simulink model "param_monitor"  (R2021a)
settings: Solver=VariableStepAuto  StartTime=0.0  StopTime=10.0  RelTol=1e-3
values from neighbouring files (symbols this model uses):
  sys_regs = 1    [motor_data.sldd]
settings Model: DataDictionary=motor_data.sldd  Creator=Litao  LastModifiedBy=Litao

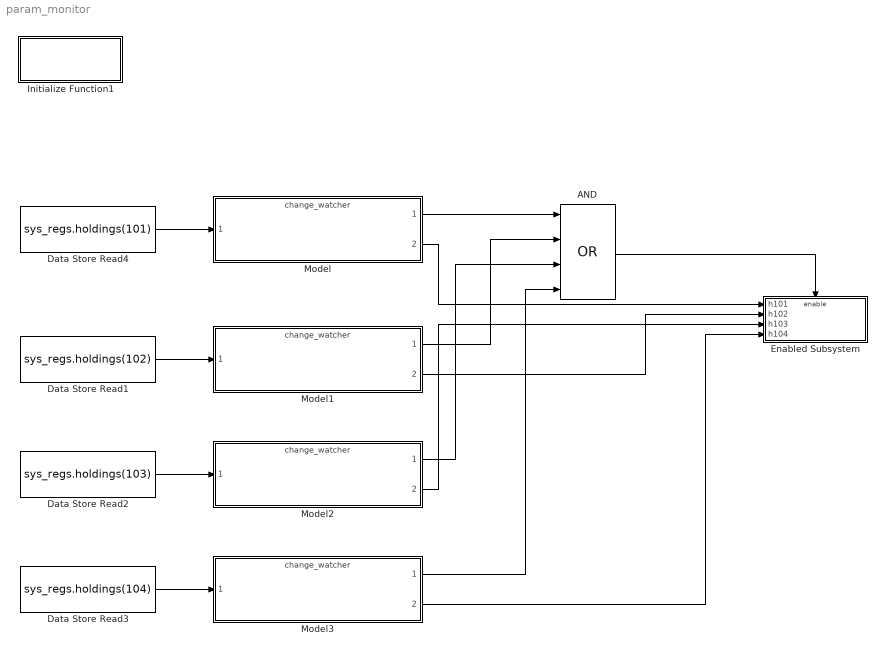
== system param_monitor ==
  AND : Logic  Operator=OR  Inputs=4  AllPortsSameDT=off  OutDataTypeStr=boolean
  Data Store Read1 : DataStoreRead  DataStoreName=sys_regs  DataStoreElements=sys_regs.holdings(102)  IndexOptions=Index vector (dialog)  Indices=1  OutputSizes=1
  Data Store Read2 : DataStoreRead  DataStoreName=sys_regs  DataStoreElements=sys_regs.holdings(103)  IndexOptions=Index vector (dialog)  Indices=1  OutputSizes=1
  Data Store Read3 : DataStoreRead  DataStoreName=sys_regs  DataStoreElements=sys_regs.holdings(104)  IndexOptions=Index vector (dialog)  Indices=1  OutputSizes=1
  Data Store Read4 : DataStoreRead  DataStoreName=sys_regs  DataStoreElements=sys_regs.holdings(101)  IndexOptions=Index vector (dialog)  Indices=1  OutputSizes=1
  Enabled Subsystem : Subsystem  TreatAsAtomicUnit=on
  Initialize Function1 : Subsystem  TreatAsAtomicUnit=on
  Model{,1..3} (4 alike) : ModelReference  ModelNameDialog=change_watcher.slx  SimulationMode=Normal  ModelReferenceVersion=1.4
  wires:
  Data Store Read4/1 -> Model/1
  AND/1 -> Enabled Subsystem/Enable
  Model/1 -> AND/1
  Model1/1 -> AND/2
  Data Store Read1/1 -> Model1/1
  Model2/1 -> AND/3
  Data Store Read2/1 -> Model2/1
  Model3/1 -> AND/4
  Data Store Read3/1 -> Model3/1
  Model/2 -> Enabled Subsystem/1(h101)
  Model1/2 -> Enabled Subsystem/2(h102)
  Model2/2 -> Enabled Subsystem/3(h103)
  Model3/2 -> Enabled Subsystem/4(h104)

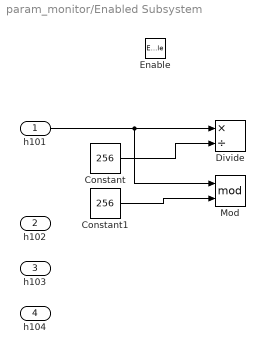
== system param_monitor/Enabled Subsystem ==
  h101 : Inport
  h102 : Inport  Port=2
  h103 : Inport  Port=3
  h104 : Inport  Port=4
  Enable : EnablePort
  Constant : Constant  Value=256
  Constant1 : Constant  Value=256
  Divide : Product  Inputs=*/
  Mod : Math  Operator=mod  SaturateOnIntegerOverflow=on
  wires:
  h101/1 -> Mod/1, Divide/1
  Constant/1 -> Divide/2
  Constant1/1 -> Mod/2

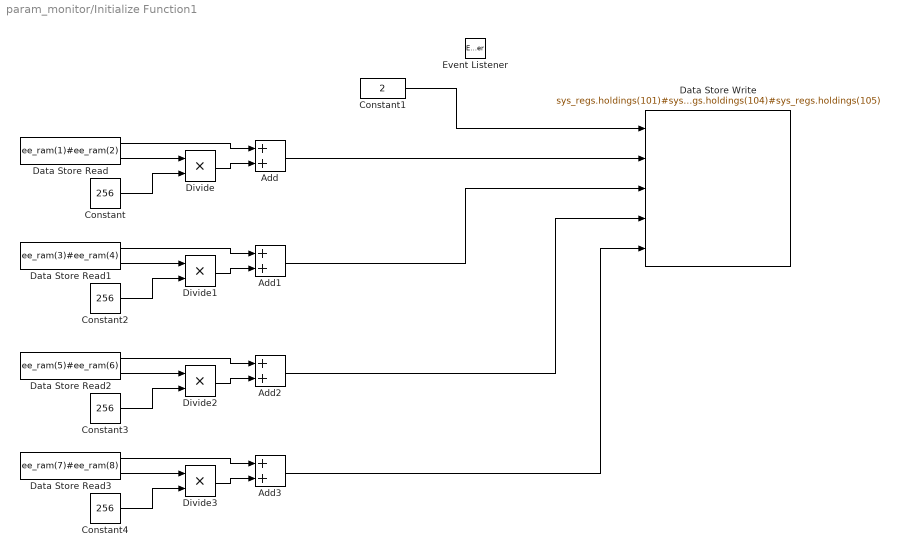
== system param_monitor/Initialize Function1 ==
  Add{,1..3} (4 alike) : Sum  AccumDataTypeStr=int16
  Constant{,2..4} (4 alike) : Constant  Value=256  OutDataTypeStr=int16
  Constant1 : Constant  Value=2  OutDataTypeStr=int16
  Data Store Read : DataStoreRead  DataStoreName=ee_ram  DataStoreElements=ee_ram(1)#ee_ram(2)  IndexOptions=Index vector (dialog)  Indices=1  OutputSizes=1
  Data Store Read1 : DataStoreRead  DataStoreName=ee_ram  DataStoreElements=ee_ram(3)#ee_ram(4)  IndexOptions=Index vector (dialog)  Indices=1  OutputSizes=1
  Data Store Read2 : DataStoreRead  DataStoreName=ee_ram  DataStoreElements=ee_ram(5)#ee_ram(6)  IndexOptions=Index vector (dialog)  Indices=1  OutputSizes=1
  Data Store Read3 : DataStoreRead  DataStoreName=ee_ram  DataStoreElements=ee_ram(7)#ee_ram(8)  IndexOptions=Index vector (dialog)  Indices=1  OutputSizes=1
  Data Store Write : DataStoreWrite  DataStoreName=sys_regs  DataStoreElements=sys_regs.holdings(101)#sys_regs.holdings(102)#sys_regs.holdings(103)#sys_regs.holdings(104)#sys_regs.holdings(105)  IndexOptions=Index vector (dialog)  Indices=1  OutputSizes=1
  Divide{,1..3} (4 alike) : Product  Inputs=**  OutDataTypeStr=int16
  Event Listener : EventListener  DisableCoverage=on  EventName=reset
  wires:
  Constant1/1 -> Data Store Write/1
  Add/1 -> Data Store Write/2
  Constant/1 -> Divide/2
  Data Store Read/2 -> Divide/1
  Data Store Read/1 -> Add/1
  Divide/1 -> Add/2
  Data Store Read1/2 -> Divide1/1
  Data Store Read1/1 -> Add1/1
  Constant2/1 -> Divide1/2
  Divide1/1 -> Add1/2
  Data Store Read2/1 -> Add2/1
  Divide2/1 -> Add2/2
  Constant3/1 -> Divide2/2
  Data Store Read2/2 -> Divide2/1
  Data Store Read3/1 -> Add3/1
  Divide3/1 -> Add3/2
  Constant4/1 -> Divide3/2
  Data Store Read3/2 -> Divide3/1
  Add1/1 -> Data Store Write/3
  Add2/1 -> Data Store Write/4
  Add3/1 -> Data Store Write/5
